simulink model "encoder_parametro_ThetaP"  (R2012b)
settings: Solver=ode45  StartTime=0.0  StopTime=10.0  RelTol=1e-3
libraries: simulink x1
settings Model: Creator=Juliano  LastModifiedBy=Juliano

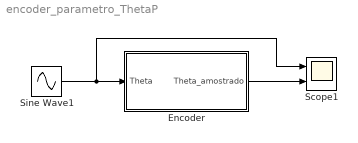
== system encoder_parametro_ThetaP ==
  Encoder : Subsystem  mask{Theta_p=5}
  Scope1 : Scope  NumInputPorts=2
      settings: YMin=150~0  YMax=575~375
  Sine Wave1 : Sin  Amplitude=360  SampleTime=0
  wires:
  Encoder/1(Theta_amostrado) -> Scope1/2
  Sine Wave1/1 -> Encoder/1(Theta), Scope1/1

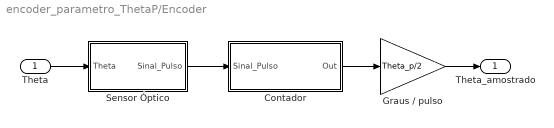
== system encoder_parametro_ThetaP/Encoder ==
  Theta : Inport
  Contador : Subsystem
  Graus / pulso : Gain  Gain=Theta_p/2
  Sensor Óptico : Subsystem
  Theta_amostrado : Outport
  wires:
  Contador/1(Out) -> Graus / pulso/1
  Sensor Óptico/1(Sinal_Pulso) -> Contador/1(Sinal_Pulso)
  Theta/1 -> Sensor Óptico/1(Theta)
  Graus / pulso/1 -> Theta_amostrado/1

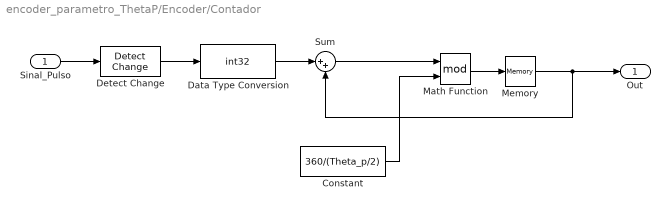
== system encoder_parametro_ThetaP/Encoder/Contador ==
  Sinal_Pulso : Inport
  Constant : Constant  Value=360/(Theta_p/2)
  Data Type Conversion : DataTypeConversion  OutDataTypeStr=int32
  Detect Change : simulink/Logic and Bit Operations/Detect Change  vinit=0  InputProcessing=Inherited  OutDataTypeStr=boolean
  Math Function : Math  Operator=mod  SaturateOnIntegerOverflow=on
  Memory : Memory
  Sum : Sum  Inputs=|++
  Out : Outport
  wires:
  Sinal_Pulso/1 -> Detect Change/1
  Memory/1 -> Out/1, Sum/2
  Constant/1 -> Math Function/2
  Detect Change/1 -> Data Type Conversion/1
  Data Type Conversion/1 -> Sum/1
  Math Function/1 -> Memory/1
  Sum/1 -> Math Function/1

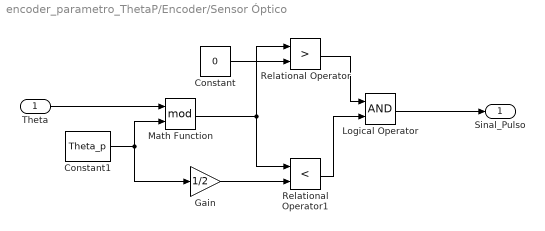
== system encoder_parametro_ThetaP/Encoder/Sensor Óptico ==
  Theta : Inport
  Constant : Constant  Value=0
  Constant1 : Constant  Value=Theta_p
  Gain : Gain  Gain=1/2
  Logical Operator : Logic  AllPortsSameDT=off  OutDataTypeStr=boolean
  Math Function : Math  Operator=mod  SaturateOnIntegerOverflow=on
  Relational Operator : RelationalOperator  Operator=>  OutDataTypeStr=boolean
  Relational Operator1 : RelationalOperator  Operator=<  OutDataTypeStr=boolean
  Sinal_Pulso : Outport
  wires:
  Math Function/1 -> Relational Operator1/1, Relational Operator/1
  Theta/1 -> Math Function/1
  Relational Operator/1 -> Logical Operator/1
  Relational Operator1/1 -> Logical Operator/2
  Constant/1 -> Relational Operator/2
  Constant1/1 -> Gain/1, Math Function/2
  Gain/1 -> Relational Operator1/2
  Logical Operator/1 -> Sinal_Pulso/1
